simulink model "Simulated_model"  (R2024a)
settings: Solver=VariableStepAuto  StartTime=0.0  StopTime=10.0  RelTol=1e-3
values from neighbouring files (symbols this model uses):
  A = [-1.064 1.000; 290.26 0.00]    [Effect_of_Q.m]    (also in LQR.m; LQR_PI.m; PD_drd.m = [-0.0089  -0.1474     0   -9.75; Pure_LQR.m = [-1.064   1.000)
  B = [-0.25; -331.40]    [Effect_of_Q.m]    (also in LQR.m; LQR_PI.m; PD_drd.m = [0; Pure_LQR.m = [-0.25)
  C = [-123.34 0.00; 0.00 1.00]    [Effect_of_Q.m]    (also in LQR.m; LQR_PI.m; PD_drd.m = eye(4); Pure_LQR.m = [-123.34   0.00)
  D = [0; 0]    [Effect_of_Q.m]    (also in LQR.m; LQR_PI.m; PD_drd.m = zeros(4,1); Pure_LQR.m = [-13.51)
  K = dlqr(Ad, Bd, Q, R)    [LQR.m]    (also in StateFeedbackController.m = K_aug(1:2); run_missile_controller.m = K_aug(1:2))
undefined symbols (not defined in the file or in its folder): dt1, dt2, L
libraries: simulink x2
settings Model: Creator=Siddarth  LastModifiedBy=Siddarth

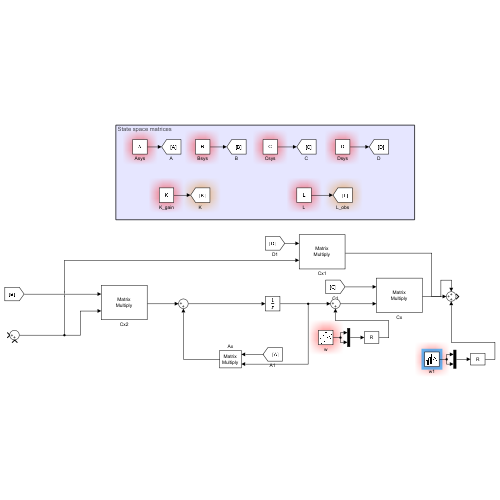
[thumbnail: Simulink's stored preview of the top-level diagram]
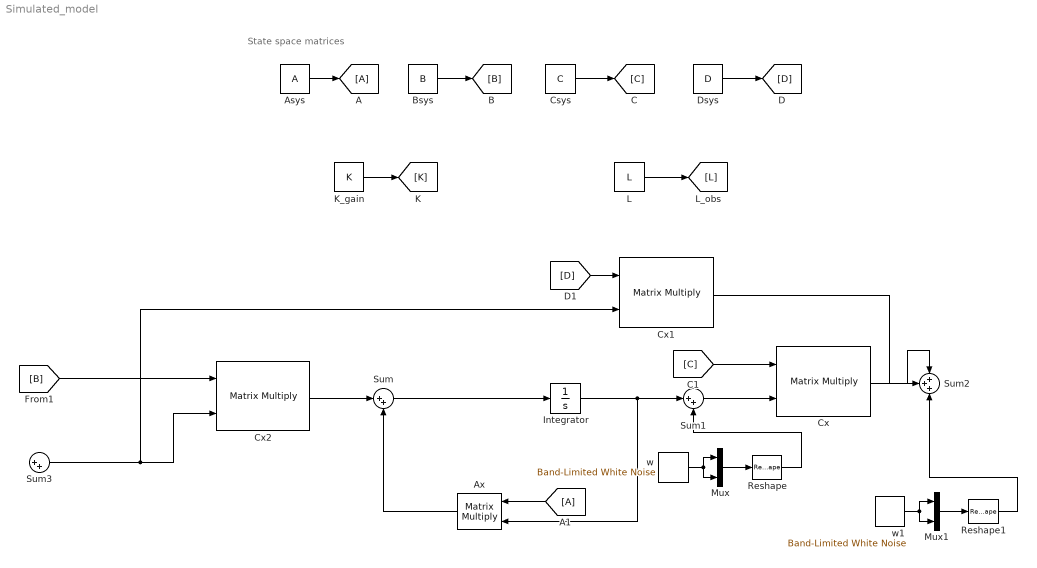
== system Simulated_model ==
  note: State space matrices
  A : Goto
  A1 : From
  Asys : Constant  Value=A
  Ax : Product  Multiplication=Matrix(*)
  Bsys : Constant  Value=B
  Csys : Constant  Value=C
  Cx : Product  Multiplication=Matrix(*)
  Cx1 : Product  Multiplication=Matrix(*)
  Cx2 : Product  Multiplication=Matrix(*)
  Dsys : Constant  Value=D
  Integrator : Integrator
  K_gain : Constant  Value=K
  L : Constant  Value=L
  Mux : Mux  Inputs=2
  Mux1 : Mux  Inputs=2
  Reshape : Reshape  OutputDimensionality=Customize  OutputDimensions=[2,1]
  Reshape1 : Reshape  OutputDimensionality=Customize  OutputDimensions=[2,1]
  Sum : Sum  Inputs=|++
  Sum1 : Sum  Inputs=|++
  Sum2 : Sum  Inputs=+++
  Sum3 : Sum  Inputs=|++
  w : simulink/Sources/Band-Limited White Noise  Cov=[0.0000001]  Ts=dt1  seed=[23341]
  w1 : simulink/Sources/Band-Limited White Noise  Cov=[0.0000001]  Ts=dt2  seed=[23341]
  wires:
  Asys/1 -> A/1
  Bsys/1 -> [B]
  Csys/1 -> [C]
  Dsys/1 -> [D]
  K_gain/1 -> [K]
  L/1 -> [L]
  A1/1 -> Ax/1
  Sum/1 -> Integrator/1
  Integrator/1 -> Ax/2, Sum1/1
  Sum1/1 -> Cx/2
  Ax/1 -> Sum/2
  [C] -> Cx/1
  Cx/1 -> Sum2/1
  [D] -> Cx1/1
  Cx1/1 -> Sum2/2
  [B] -> Cx2/1
  Sum3/1 -> Cx1/2, Cx2/2
  Cx2/1 -> Sum/1
  w/1 -> Mux/1, Mux/2
  Mux/1 -> Reshape/1
  Reshape/1 -> Sum1/2
  Reshape1/1 -> Sum2/3
  Mux1/1 -> Reshape1/1
  w1/1 -> Mux1/1, Mux1/2
